simulink model "problem2_3"  (R2020a)
settings: Solver=VariableStepAuto  StartTime=0.0  StopTime=10.0  RelTol=1e-3
settings Model: Creator=dinhm  LastModifiedBy=dinhm

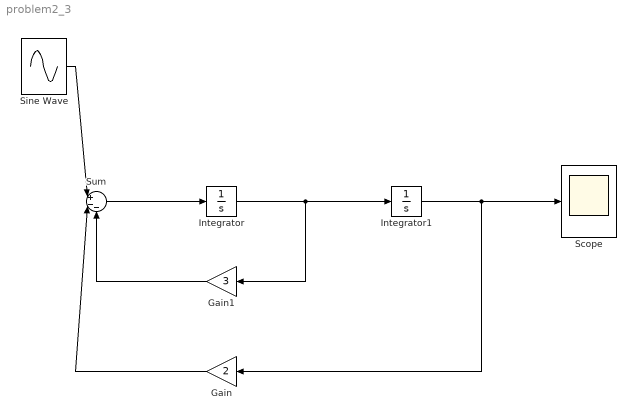
== system problem2_3 ==
  Gain : Gain  Gain=2
  Gain1 : Gain  Gain=3
  Integrator : Integrator
  Integrator1 : Integrator
  Scope : Scope
  Sine Wave : Sin  Amplitude=5  Phase=pi/4  SampleTime=0
  Sum : Sum  Inputs=|+--
  wires:
  Sine Wave/1 -> Sum/1
  Gain1/1 -> Sum/3
  Gain/1 -> Sum/2
  Sum/1 -> Integrator/1
  Integrator/1 -> Gain1/1, Integrator1/1
  Integrator1/1 -> Scope/1, Gain/1
